simulink model "Solar_tied_SAPF"  (R2015a)
settings: Solver=ode45  StartTime=0.0  StopTime=.2  RelTol=1e-3
libraries: powerlib x30, dsparch4 x1, re_lib x1, powerlib_extras x1
settings Model: Creator=Mahbub  LastModifiedBy=Mahbub

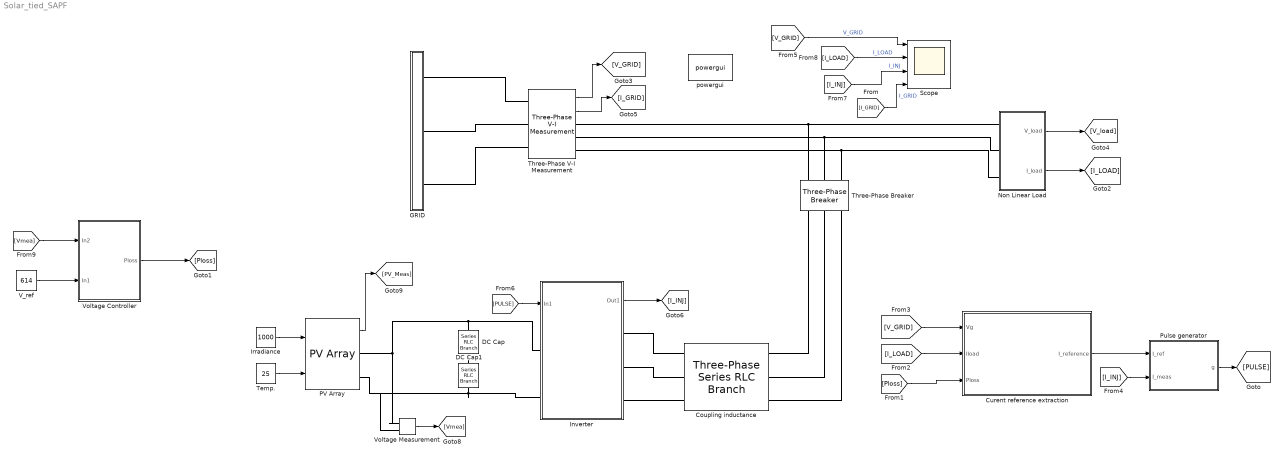
== system Solar_tied_SAPF ==
  "Coupling inductance " : powerlib/Elements/Three-Phase Series RLC Branch  LConnTagsString=A|B|C  RConnTagsString=A|B|C  BranchType=L  Resistance=.001  Inductance=1.2e-3  Capacitance=1e-6  Measurements=None
  "Curent reference extraction " : Subsystem
  DC Cap : powerlib/Elements/Series RLC Branch  LConnTagsString=__new0  RConnTagsString=__new0  BranchType=C  Resistance=1  Inductance=1e-3  SetiL0=off  InitialCurrent=0  Capacitance=40e-6  Setx0=off  InitialVoltage=400  Measurements=None
  DC Cap1 : powerlib/Elements/Series RLC Branch  LConnTagsString=__new0  RConnTagsString=__new0  BranchType=C  Resistance=1  Inductance=1e-3  SetiL0=off  InitialCurrent=0  Capacitance=40e-6  Setx0=off  InitialVoltage=400  Measurements=None
  "GRID " : Subsystem
  "Inverter " : Subsystem
  Irradiance : Constant  Value=1000
  Non Linear Load : Subsystem
  PV Array : re_lib/Solar/PV Array  Npar=5  Nser=20  PlotType=array @ 1000 W/m2 & specified temperatures  S_vec="[ 1000  500  100 ]"  Temp_C_vec="[ 45 25  ]"  ModuleName=1Soltech 1STH-250-WH  PlotWhenSelected=off  Pm=250.205  Ncell=60  Voc=37.3  Isc=8.66  Vm=30.7  Im=8.15  beta_Voc_pc=-0.36901  alpha_Isc_pc=0.086998  beta_Voc=-0.13764  alpha_Isc=0.007534  IL=8.7106  I0=4.1601e-10  nI=1.019  Rsh=224.1886  Rs=0.23724  BAL=off  Tc=1e-6  Tfilter=5e-5
      settings: AttributesFormatString=|
      | %<ModuleName>
      | %<Nser>-module string
      | %<Npar> parallel strings
  Pulse generator : Subsystem
  Scope : Scope  NumInputPorts=4
      settings: ShowLegends=on  TimeRange=0.06664500000000001  YMin=-400~-100~-40~-100  YMax=400~100~40~100  SaveName=ScopeData3
  "Temp. " : Constant  Value=25
  Three-Phase V-I Measurement : powerlib/Measurements/Three-Phase V-I Measurement  VoltageMeasurement=phase-to-ground  SetLabelV=off  LabelV=Vabc  Vpu=off  VpuLL=off  CurrentMeasurement=yes  SetLabelI=off  LabelI=Iabc  Ipu=off  Pbase=100e6  Vbase=500e3  OutputType=Complex  PhasorSimulation=off  PSBequivalent=0
  Three-Phase Breaker : powerlib/Elements/Three-Phase Breaker  InitialState=open  SwitchA=on  SwitchB=on  SwitchC=on  SwitchTimes=0.01  External=off  BreakerResistance=1e-6  SnubberResistance=1e6  SnubberCapacitance=inf  Measurements=None
  "V_ref " : Constant  Value=614
  "Voltage Controller " : Subsystem
  Voltage Measurement : powerlib/Measurements/Voltage Measurement  PhasorSimulation=off  OutputType=Complex  PSBequivalent=0
  powergui : powerlib/powergui  Priority=1  SimulationMode=Discrete  SolverType=Tustin/Backward Euler (TBE)  SampleTime=5e-6  frequency=60  SPID=off  DisableSnubberDevices=off  DisableRonSwitches=off  DisableVfSwitches=off  SwTol=0  DisplayEquations=off  Interpol=off  methode=off  Ts=100  FunctionMessages=off  echomessages=off  HookPort=off  EnableUseOfTLC=off  x0status=blocks  frequencyindice=50  Pbase=100e6  ErrMax=1e-4  Iterations=50  UnitsV=kV  UnitsW=MW  buscounter=0  RestoreLinks=warning  ResistiveCurrentMeasurement=off  Frange=[0:2:500]  Ylog=off  Xlog=on  ShowGrid=off  save=off  variable=ZData  structure=ScopeData3  ZoomFFT=off  StartTime=.02  cycles=2  DisplayStyle=1  fundamental=60  FreqAxis=off  MaxFrequency=1000  frequencyindicesteady=1  RmsSteady=1  display=off
  wires:
  "Curent reference extraction "/1(I_reference) -> Pulse generator/1(I_ref)
  Pulse generator/1(g) -> [PULSE]
  "Voltage Controller "/1("Ploss ") -> [Ploss]
  [Ploss] -> "Curent reference extraction "/3("Ploss ")
  [I_LOAD] -> "Curent reference extraction "/2(Iload)
  Three-Phase V-I Measurement/1 -> [V_GRID]
  [V_GRID] -> "Curent reference extraction "/1("Vg ")
  [I_INJ] -> Pulse generator/2(I_meas)
  Non Linear Load/1(V_load) -> [V_load]
  Three-Phase V-I Measurement/2 -> [I_GRID]
  "Inverter "/1(Out1) -> [I_INJ]
  [PULSE] -> "Inverter "/1(In1)
  [V_GRID] -> Scope/1  "V_GRID"
  Non Linear Load/2(I_load) -> [I_LOAD]
  "Temp. "/1 -> PV Array/2
  Irradiance/1 -> PV Array/1
  [Vmea] -> "Voltage Controller "/1(In2)
  Voltage Measurement/1 -> [Vmea]
  PV Array/1 -> [PV_Meas]
  "V_ref "/1 -> "Voltage Controller "/2(In1)
  [I_LOAD] -> Scope/2  "I_LOAD"
  [I_GRID] -> Scope/4  "I_GRID"
  [I_INJ] -> Scope/3  "I_INJ"
  connections:
  Three-Phase Breaker/LConn1 -- Three-Phase V-I Measurement/RConn1 -- Non Linear Load/LConn1
  Three-Phase V-I Measurement/RConn2 -- Non Linear Load/LConn2 -- Three-Phase Breaker/LConn2
  Three-Phase Breaker/LConn3 -- Three-Phase V-I Measurement/RConn3 -- Non Linear Load/LConn3
  "Coupling inductance "/RConn1 -- Three-Phase Breaker/RConn1
  "Coupling inductance "/RConn2 -- Three-Phase Breaker/RConn2
  "Coupling inductance "/RConn3 -- Three-Phase Breaker/RConn3
  "Coupling inductance "/LConn1 -- "Inverter "/RConn1
  "Coupling inductance "/LConn2 -- "Inverter "/RConn2
  "Coupling inductance "/LConn3 -- "Inverter "/RConn3
  DC Cap/RConn1 -- DC Cap1/LConn1
  "Inverter "/LConn1 -- Voltage Measurement/LConn1 -- PV Array/RConn1 -- DC Cap/LConn1
  DC Cap1/RConn1 -- PV Array/RConn2 -- Voltage Measurement/LConn2 -- "Inverter "/LConn2
  Three-Phase V-I Measurement/LConn1 -- "GRID "/RConn1
  Three-Phase V-I Measurement/LConn2 -- "GRID "/RConn2
  Three-Phase V-I Measurement/LConn3 -- "GRID "/RConn3

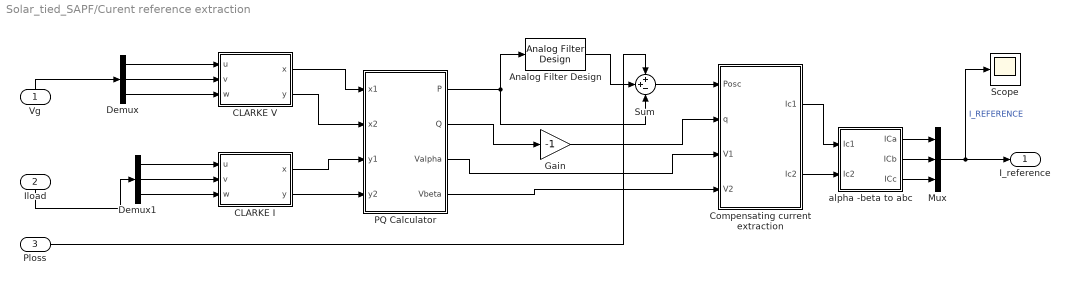
== system Solar_tied_SAPF/Curent reference extraction  ==
  "Vg " : Inport
  Iload : Inport  Port=2
  "Ploss " : Inport  Port=3
  Analog Filter Design : dsparch4/Analog Filter Design  method=Butterworth  filttype=Lowpass  N=5  Wlo=2*pi*50  Whi=80  Rp=2  Rs=40
  CLARKE I : MATLAB Function  TreatAsAtomicUnit=on
  CLARKE V : MATLAB Function  TreatAsAtomicUnit=on
  "Compensating current extraction " : MATLAB Function  TreatAsAtomicUnit=on
  Demux : Demux  Outputs=3
  Demux1 : Demux  Outputs=3
  Gain : Gain  Gain=-1
  Mux : Mux  Inputs=3
  PQ Calculator : MATLAB Function  TreatAsAtomicUnit=on
  Scope : Scope
      settings: YMin=-30  YMax=30  SaveName=ScopeData2
  Sum : Sum  Inputs=++-
  "alpha -beta to abc " : MATLAB Function  TreatAsAtomicUnit=on
  I_reference : Outport
  wires:
  PQ Calculator/1(P) -> Sum/3, Analog Filter Design/1
  CLARKE V/1(x) -> PQ Calculator/1(x1)
  Sum/1 -> "Compensating current extraction "/1(Posc)
  PQ Calculator/3(Valpha) -> "Compensating current extraction "/3(V1)
  CLARKE I/1(x) -> PQ Calculator/3(y1)
  "Compensating current extraction "/1(Ic1) -> "alpha -beta to abc "/1(Ic1)
  CLARKE V/2(y) -> PQ Calculator/2(x2)
  CLARKE I/2(y) -> PQ Calculator/4(y2)
  Demux/3 -> CLARKE V/3(w)
  "alpha -beta to abc "/3(ICc) -> Mux/3
  Mux/1 -> Scope/1, I_reference/1  "I_REFERENCE"
  "Vg "/1 -> Demux/1
  Iload/1 -> Demux1/1
  Demux/2 -> CLARKE V/2(v)
  Demux1/3 -> CLARKE I/3(w)
  "Ploss "/1 -> Sum/1
  "Compensating current extraction "/2(Ic2) -> "alpha -beta to abc "/2(Ic2)
  "alpha -beta to abc "/2(ICb) -> Mux/2
  Demux1/1 -> CLARKE I/1(u)
  Demux1/2 -> CLARKE I/2(v)
  Demux/1 -> CLARKE V/1(u)
  "alpha -beta to abc "/1(ICa) -> Mux/1
  Analog Filter Design/1 -> Sum/2
  PQ Calculator/4(Vbeta) -> "Compensating current extraction "/4(V2)
  PQ Calculator/2(Q) -> Gain/1
  Gain/1 -> "Compensating current extraction "/2(q)

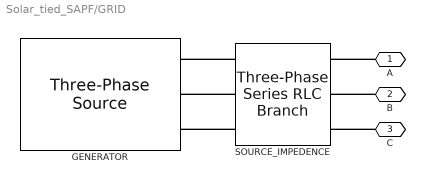
== system Solar_tied_SAPF/GRID  ==
  "GENERATOR " : powerlib/Electrical Sources/Three-Phase Source  Voltage=400  PhaseAngle=0  Frequency=50  InternalConnection=Yg  SpecifyImpedance=off  Resistance=0.001  Inductance=1e-8  ShortCircuitLevel=100e6  BaseVoltage=25e3  XRratio=7  BusType=swing  Pref=0  Qref=0  Qmin=-inf  Qmax=inf
  SOURCE_IMPEDENCE : powerlib/Elements/Three-Phase Series RLC Branch  LConnTagsString=A|B|C  RConnTagsString=A|B|C  BranchType=RL  Resistance=.01  Inductance=1e-6  Capacitance=1e-6  Measurements=None
  A : PMIOPort  Port=1  Side=Right
  B : PMIOPort  Port=2  Side=Right
  C : PMIOPort  Port=3  Side=Right
  connections:
  SOURCE_IMPEDENCE/LConn2 -- "GENERATOR "/RConn2
  SOURCE_IMPEDENCE/LConn3 -- "GENERATOR "/RConn3
  SOURCE_IMPEDENCE/LConn1 -- "GENERATOR "/RConn1
  B/RConn1 -- SOURCE_IMPEDENCE/RConn2
  A/RConn1 -- SOURCE_IMPEDENCE/RConn1
  C/RConn1 -- SOURCE_IMPEDENCE/RConn3

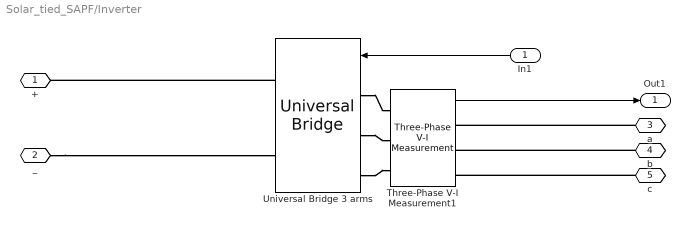
== system Solar_tied_SAPF/Inverter  ==
  In1 : Inport
  Three-Phase V-I Measurement1 : powerlib/Measurements/Three-Phase V-I Measurement  VoltageMeasurement=no  SetLabelV=off  LabelV=Vabc  Vpu=off  VpuLL=off  CurrentMeasurement=yes  SetLabelI=off  LabelI=Iabc  Ipu=off  Pbase=100e6  Vbase=500e3  OutputType=Complex  PhasorSimulation=off  PSBequivalent=0
  Universal Bridge 3 arms : powerlib/Power Electronics/Universal Bridge  Arms=3  SnubberResistance=10000  SnubberCapacitance=inf  Device=IGBT / Diodes  Ron=1e-4  Lon=0  ForwardVoltages="[  1  1  ]"  ForwardVoltage=.8  GTOparameters=[ 10e-6 , 20e-6 ]  IGBTparameters=[ 1e-6 , 2e-6 ]  Measurements=None  Measurements_2=None  converterType=Rectifier
  + : PMIOPort  Port=1  Side=Left
  _ : PMIOPort  Port=2  Side=Left
  a : PMIOPort  Port=3  Side=Right
  b : PMIOPort  Port=4  Side=Right
  c : PMIOPort  Port=5  Side=Right
  Out1 : Outport
  wires:
  Three-Phase V-I Measurement1/1 -> Out1/1
  In1/1 -> Universal Bridge 3 arms/1
  connections:
  b/RConn1 -- Three-Phase V-I Measurement1/RConn2
  _/RConn1 -- Universal Bridge 3 arms/RConn2
  Universal Bridge 3 arms/LConn3 -- Three-Phase V-I Measurement1/LConn3
  a/RConn1 -- Three-Phase V-I Measurement1/RConn1
  Universal Bridge 3 arms/LConn2 -- Three-Phase V-I Measurement1/LConn2
  c/RConn1 -- Three-Phase V-I Measurement1/RConn3
  Universal Bridge 3 arms/LConn1 -- Three-Phase V-I Measurement1/LConn1
  Universal Bridge 3 arms/RConn1 -- +/RConn1

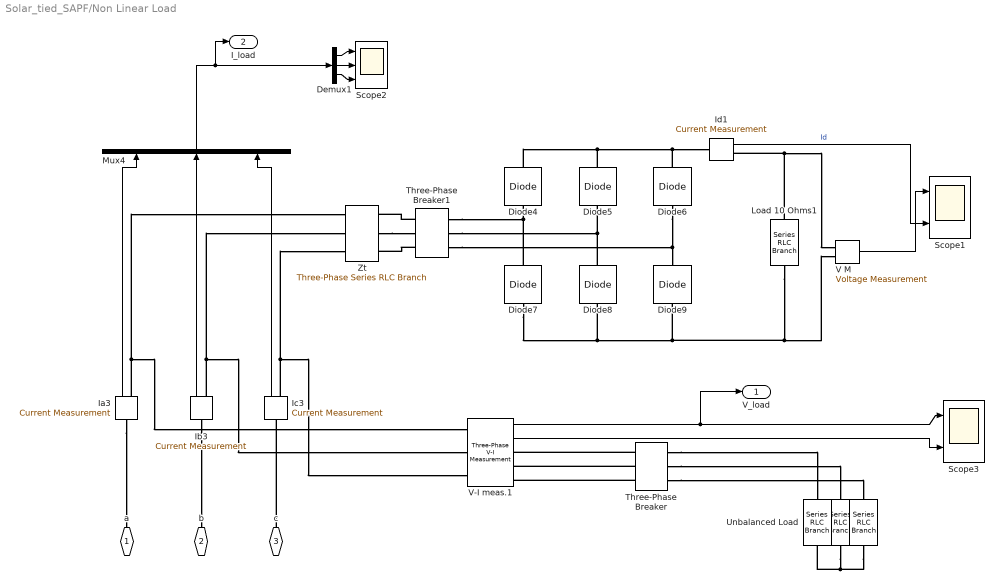
== system Solar_tied_SAPF/Non Linear Load ==
  " " : powerlib/Elements/Series RLC Branch  LConnTagsString=__new0  RConnTagsString=__new0  BranchType=R  Resistance=4  Inductance=[]  SetiL0=off  InitialCurrent=0  Capacitance=[]  Setx0=off  InitialVoltage=0  Measurements=None
  "   " : powerlib/Elements/Series RLC Branch  LConnTagsString=__new0  RConnTagsString=__new0  BranchType=R  Resistance=6  Inductance=[]  SetiL0=off  InitialCurrent=0  Capacitance=[]  Setx0=off  InitialVoltage=0  Measurements=None
  Demux1 : Demux  Outputs=3
  Diode{4..9} (6 alike) : powerlib/Power Electronics/Diode  Ron=1e-1  Lon=0  Vf=0.8  IC=0  UseSnubber=off  Rs=1000  Cs=0.1e-6  Measurements=off
  Ia3 : powerlib/Measurements/Current Measurement  PhasorSimulation=off  OutputType=Complex  PSBequivalent=0
  Ib3 : powerlib/Measurements/Current Measurement  PhasorSimulation=off  OutputType=Complex  PSBequivalent=0
  Ic3 : powerlib/Measurements/Current Measurement  PhasorSimulation=off  OutputType=Complex  PSBequivalent=0
  Id1 : powerlib/Measurements/Current Measurement  Tag=PoWeRsYsTeMmEaSuReMeNt  PhasorSimulation=off  OutputType=Magnitude  PSBequivalent=0
  Load 10 Ohms1 : powerlib/Elements/Series RLC Branch  LConnTagsString=__new0  RConnTagsString=__new0  BranchType=R  Resistance=10  Inductance=[]  SetiL0=off  InitialCurrent=0  Capacitance=[]  Setx0=off  InitialVoltage=0  Measurements=None
  Mux4 : Mux  Inputs=3
  Scope1 : Scope  NumInputPorts=2
      settings: TimeRange=0.1  YMin=210~4.2  YMax=245~4.9  DataFormat=Structure
  Scope2 : Scope  NumInputPorts=3
      settings: TimeRange=0.1  YMin=0~-56.5~-5  YMax=60~-48~60  SaveName=psb3phPWM1_str8  MaxDataPoints=500000
  Scope3 : Scope  NumInputPorts=2
      settings: TimeRange=0.1  YMin=-350~-70  YMax=350~110  DataFormat=Structure
  Three-Phase Breaker : powerlib/Elements/Three-Phase Breaker  InitialState=open  SwitchA=on  SwitchB=on  SwitchC=on  SwitchTimes=0.2  External=off  BreakerResistance=1e-5  SnubberResistance=1e6  SnubberCapacitance=inf  Measurements=None
  Three-Phase Breaker1 : powerlib/Elements/Three-Phase Breaker  InitialState=open  SwitchA=on  SwitchB=on  SwitchC=on  SwitchTimes=0  External=off  BreakerResistance=1e-5  SnubberResistance=1e6  SnubberCapacitance=inf  Measurements=None
  Unbalanced Load : powerlib/Elements/Series RLC Branch  LConnTagsString=__new0  RConnTagsString=__new0  BranchType=R  Resistance=2  Inductance=[]  SetiL0=off  InitialCurrent=0  Capacitance=[]  Setx0=off  InitialVoltage=0  Measurements=None
  V M : powerlib/Measurements/Voltage Measurement  PhasorSimulation=off  OutputType=Complex  PSBequivalent=0
  V-I meas.1 : powerlib/Measurements/Three-Phase V-I Measurement  VoltageMeasurement=phase-to-ground  SetLabelV=off  LabelV=Vabc  Vpu=off  VpuLL=off  CurrentMeasurement=yes  SetLabelI=off  LabelI=Iabc  Ipu=off  Pbase=100e6  Vbase=500e3  OutputType=Complex  PhasorSimulation=off  PSBequivalent=0
  Zt : powerlib/Elements/Three-Phase Series RLC Branch  LConnTagsString=A|B|C  RConnTagsString=A|B|C  BranchType=RL  Resistance=0.001  Inductance=1e-6  Capacitance=1e-6  Measurements=None
  a : PMIOPort  Port=1  Side=Left
  b : PMIOPort  Port=2  Side=Left
  c : PMIOPort  Port=3  Side=Left
  V_load : Outport
  I_load : Outport  Port=2
  wires:
  Mux4/1 -> I_load/1, Demux1/1
  Demux1/2 -> Scope2/2
  Demux1/3 -> Scope2/3
  Demux1/1 -> Scope2/1
  V M/1 -> Scope1/1
  Id1/1 -> Scope1/2  "Id"
  V-I meas.1/1 -> Scope3/1, V_load/1
  V-I meas.1/2 -> Scope3/2
  Ic3/1 -> Mux4/3
  Ib3/1 -> Mux4/2
  Ia3/1 -> Mux4/1
  connections:
  Ia3/LConn1 -- a/RConn1
  Ib3/LConn1 -- b/RConn1
  Ic3/RConn1 -- V-I meas.1/LConn3 -- Zt/LConn3
  Ib3/RConn1 -- V-I meas.1/LConn2 -- Zt/LConn2
  Ia3/RConn1 -- V-I meas.1/LConn1 -- Zt/LConn1
  Diode6/RConn1 -- Id1/LConn1 -- Diode4/RConn1 -- Diode5/RConn1
  Load 10 Ohms1/LConn1 -- Id1/RConn1 -- V M/LConn1
  Diode9/LConn1 -- Diode7/LConn1 -- Diode8/LConn1 -- V M/LConn2 -- Load 10 Ohms1/RConn1
  Unbalanced Load/RConn1 -- " "/RConn1 -- "   "/RConn1
  c/RConn1 -- Ic3/LConn1
  Three-Phase Breaker/LConn3 -- V-I meas.1/RConn3
  Three-Phase Breaker/LConn2 -- V-I meas.1/RConn2
  Three-Phase Breaker/LConn1 -- V-I meas.1/RConn1
  Three-Phase Breaker/RConn1 -- Unbalanced Load/LConn1
  Three-Phase Breaker/RConn2 -- " "/LConn1
  Three-Phase Breaker/RConn3 -- "   "/LConn1
  Diode7/RConn1 -- Diode4/LConn1 -- Three-Phase Breaker1/RConn1
  Diode8/RConn1 -- Diode5/LConn1 -- Three-Phase Breaker1/RConn2
  Diode6/LConn1 -- Diode9/RConn1 -- Three-Phase Breaker1/RConn3
  Three-Phase Breaker1/LConn1 -- Zt/RConn1
  Zt/RConn2 -- Three-Phase Breaker1/LConn2
  Three-Phase Breaker1/LConn3 -- Zt/RConn3

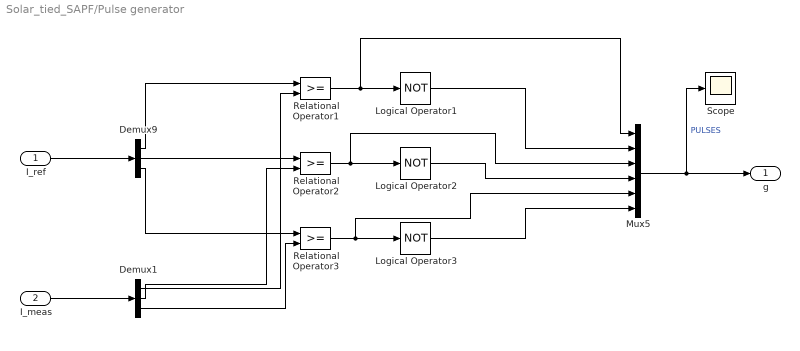
== system Solar_tied_SAPF/Pulse generator ==
  I_ref : Inport
  I_meas : Inport  Port=2
  Demux1 : Demux  Outputs=3
  Demux9 : Demux  Outputs=3
  Logical Operator1 : Logic  Operator=NOT  AllPortsSameDT=off  OutDataTypeStr=boolean
  Logical Operator2 : Logic  Operator=NOT  AllPortsSameDT=off  OutDataTypeStr=boolean
  Logical Operator3 : Logic  Operator=NOT  AllPortsSameDT=off  OutDataTypeStr=boolean
  Mux5 : Mux  Inputs=6
  Relational Operator1 : RelationalOperator  OutDataTypeStr=boolean
  Relational Operator2 : RelationalOperator  OutDataTypeStr=boolean
  Relational Operator3 : RelationalOperator  OutDataTypeStr=boolean
  Scope : Scope
      settings: SaveName=ScopeData6
  g : Outport
  wires:
  Relational Operator1/1 -> Logical Operator1/1, Mux5/1
  Relational Operator2/1 -> Logical Operator2/1, Mux5/3
  Relational Operator3/1 -> Logical Operator3/1, Mux5/5
  Demux9/1 -> Relational Operator1/1
  Demux9/3 -> Relational Operator3/1
  Logical Operator1/1 -> Mux5/2
  Logical Operator2/1 -> Mux5/4
  Logical Operator3/1 -> Mux5/6
  Mux5/1 -> Scope/1, g/1  "PULSES"
  Demux9/2 -> Relational Operator2/1
  Demux1/1 -> Relational Operator1/2
  Demux1/2 -> Relational Operator2/2
  Demux1/3 -> Relational Operator3/2
  I_ref/1 -> Demux9/1
  I_meas/1 -> Demux1/1

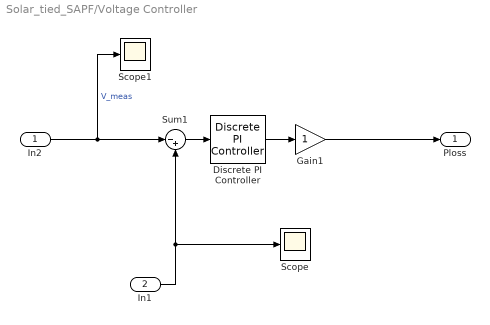
== system Solar_tied_SAPF/Voltage Controller  ==
  In2 : Inport
  In1 : Inport  Port=2
  Discrete PI Controller : powerlib_extras/Discrete  Control Blocks/Discrete PI Controller  Kp=5  Ki=2  Par_Limits=[1e6 -1e6]  Init=0  Ts=5e-6
  Gain1 : Gain
  Scope : Scope
      settings: YMin=614  YMax=614  SaveName=ScopeData4
  Scope1 : Scope
      settings: YMin=0  YMax=1000  SaveName=ScopeData5
  Sum1 : Sum  Inputs=|-+
  "Ploss " : Outport
  wires:
  Gain1/1 -> "Ploss "/1
  Discrete PI Controller/1 -> Gain1/1
  In2/1 -> Scope1/1, Sum1/1  "V_meas"
  Sum1/1 -> Discrete PI Controller/1
  In1/1 -> Scope/1, Sum1/2

== matlab function Solar_tied_SAPF/Curent reference extraction /CLARKE I ==
  data: u input; x output; v input; w input; y output
function [x,y] = VCT(u,v,w)
%#em1

x = sqrt(2/3)*(u-(0.5*v)-(0.5*w));
y = sqrt(2)*(0+(0.5*v)-(0.5*w));

== matlab function Solar_tied_SAPF/Curent reference extraction /CLARKE V ==
  data: u input; x output; v input; w input; y output
function [x,y] = VCT(u,v,w)


x = sqrt(2/3)*(u-(0.5*v)-(0.5*w));
y = sqrt(2)*(0+(0.5*v)-(0.5*w));


end

== matlab function Solar_tied_SAPF/Curent reference extraction /alpha -beta to abc  ==
  data: Ic1 input; ICa output; Ic2 input; ICb output; ICc output
function [ICa,ICb,ICc] = Ical(Ic1,Ic2)
%#em1

ICa = sqrt(2/3)*(Ic1);
ICb = sqrt(2/3)*((-0.5*Ic1)+((sqrt(3)/2)*Ic2));
ICc = sqrt(2/3)*((-0.5*Ic1)-((sqrt(3)/2)*Ic2));

== matlab function Solar_tied_SAPF/Curent reference extraction /Compensating current extraction  ==
  data: Posc input; Ic1 output; q input; V1 input; Ic2 output; V2 input
function [Ic1,Ic2] = ICOM(Posc,q,V1,V2)
%#em1

Ic1 = (-1/(V1^2 + V2^2))*((Posc*V1)+(q*V2));
Ic2 = (-1/(V1^2 + V2^2))*((Posc*V2)-(q*V1));

== matlab function Solar_tied_SAPF/Curent reference extraction /PQ Calculator ==
  data: x1 input; P output; Q output; x2 input; y1 input; y2 input; Valpha output; Vbeta output
function [P,Q,Valpha,Vbeta] = PQ(x1,x2,y1,y2)
%#em1

P = (x1*y1)+(x2*y2);
Q = (x2*y1)-(x1*y2);
Valpha = x1;
Vbeta = x2;
